simulink model "orientationandmotor"  (R2020a)
settings: Solver=VariableStepAuto  StartTime=0.0  StopTime=10.0  RelTol=1e-3
undefined symbols (not defined in the file): b, d
settings Model: Creator=Muni Kumar  LastModifiedBy=Muni Kumar

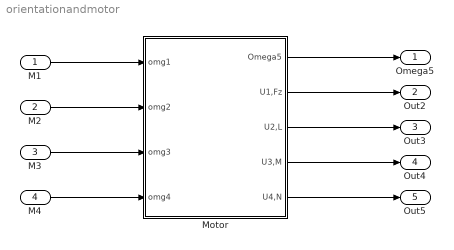
== system orientationandmotor ==
  M1 : Inport
  M2 : Inport  Port=2
  M3 : Inport  Port=3
  M4 : Inport  Port=4
  Motor : Subsystem
  Omega5 : Outport
  Out2 : Outport  Port=2  SignalName=U1,Fz
  Out3 : Outport  Port=3  SignalName=U2,L
  Out4 : Outport  Port=4  SignalName=U3,M
  Out5 : Outport  Port=5  SignalName=U4,N
  wires:
  M1/1 -> Motor/1(omg1)
  M2/1 -> Motor/2(omg2)
  M3/1 -> Motor/3(omg3)
  M4/1 -> Motor/4(omg4)
  Motor/1(Omega5) -> Omega5/1
  Motor/2(U1,Fz) -> Out2/1
  Motor/3(U2,L) -> Out3/1
  Motor/4(U3,M) -> Out4/1
  Motor/5(U4,N) -> Out5/1

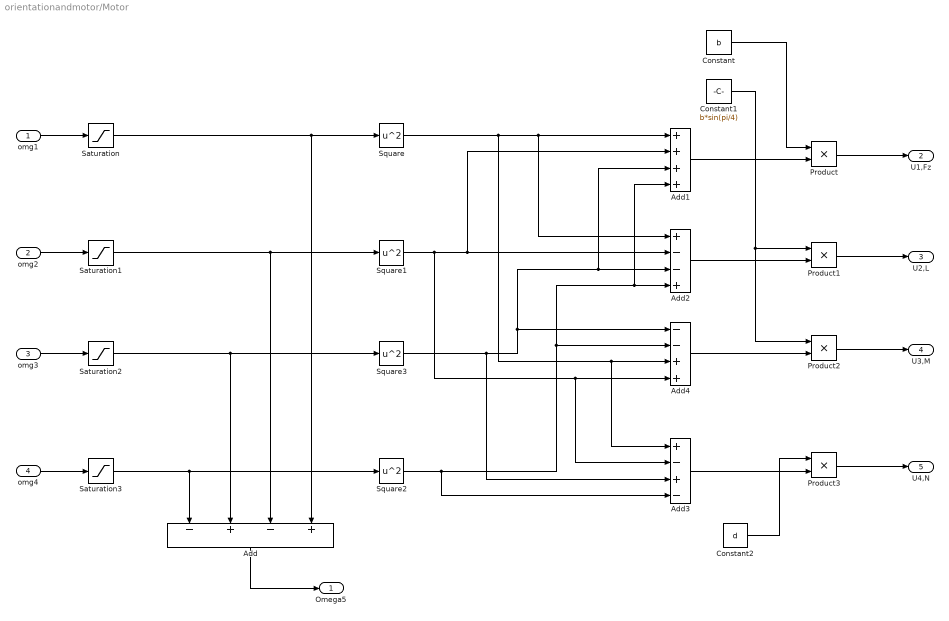
== system orientationandmotor/Motor ==
  omg1 : Inport
  omg2 : Inport  Port=2
  omg3 : Inport  Port=3
  omg4 : Inport  Port=4
  Add : Sum  Inputs=-+-+
  Add1 : Sum  Inputs=++++
  Add2 : Sum  Inputs=+--+
  Add3 : Sum  Inputs=+-+-
  Add4 : Sum  Inputs=--++
  Constant : Constant  Value=b
  Constant1 : Constant  Value=b*sin(pi/4)
  Constant2 : Constant  Value=d
  Product{,1..3} (4 alike) : Product
  Saturation{,1..3} (4 alike) : Saturate
  Square{,1..3} (4 alike) : Math  Operator=square  SaturateOnIntegerOverflow=on
  Omega5 : Outport
  U1,Fz : Outport  Port=2
  U2,L : Outport  Port=3
  U3,M : Outport  Port=4
  U4,N : Outport  Port=5
  wires:
  Product3/1 -> U4,N/1
  omg1/1 -> Saturation/1
  omg2/1 -> Saturation1/1
  Add/1 -> Omega5/1
  omg3/1 -> Saturation2/1
  Product2/1 -> U3,M/1
  Saturation/1 -> Add/4, Square/1
  Product1/1 -> U2,L/1
  Product/1 -> U1,Fz/1
  Add2/1 -> Product1/2
  Square3/1 -> Add3/3, Add4/1, Add1/3, Add2/3
  Square2/1 -> Add4/2, Add1/4, Add2/4, Add3/4
  Square/1 -> Add3/1, Add4/3, Add2/1, Add1/1
  Saturation3/1 -> Add/1, Square2/1
  Constant/1 -> Product/1
  Square1/1 -> Add3/2, Add4/4, Add1/2, Add2/2
  omg4/1 -> Saturation3/1
  Constant1/1 -> Product2/1, Product1/1
  Add4/1 -> Product2/2
  Add1/1 -> Product/2
  Add3/1 -> Product3/2
  Saturation2/1 -> Add/2, Square3/1
  Saturation1/1 -> Add/3, Square1/1
  Constant2/1 -> Product3/1
